simulink model "roachf_1024_bao"  (Simulink 7.5)
settings: Solver=ode45  StartTime=0.0  StopTime=10.0  RelTol=1e-3
undefined symbols (not defined in the file or in its folder): Down, quant, Up
libraries: xbsIndex_r4 x1081, xps_library x49, casper_library_misc x17, casper_library_delays x9, casper_library_sources x4, xbsReplacements_r4 x4, xrbsControl_r4 x1
(part 1 of 11)
settings Model: Creator=zaki  LastModifiedBy=zaki
settings DebuggingCC: StrictBusMsg=Warning

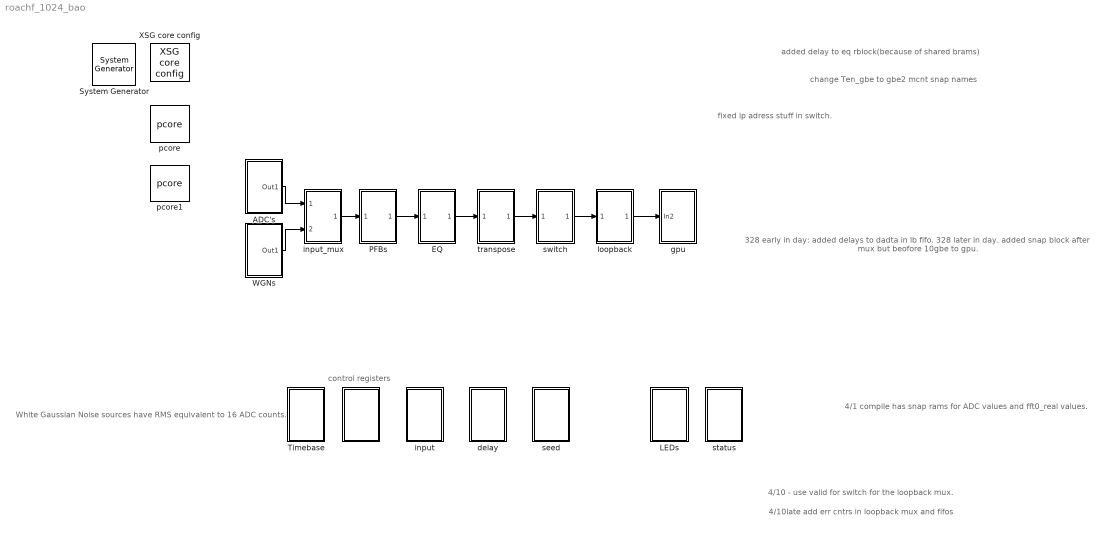
== system roachf_1024_bao ==
  note: White Gaussian Noise
      | sources have RMS
      | equivalent to 16 ADC
      | counts.
  note: fixed ip adress stuff in switch.
  note: 328 early in day: added delays to dadta in lb fifo.
      | 328 later in day. added snap block after mux but beofore
      | 10gbe to gpu.
  note: 4/1 compile has snap rams for ADC values
      | and fft0_real values.
  note: 4/10 - use valid for switch for the loopback mux.
  note: 4/10late add err cntrs in loopback mux and fifos
  note: control registers
  note: added delay to eq rblock(because of shared brams)
  note: change Ten_gbe to gbe2
      | mcnt snap names
  " " : Subsystem
  " System Generator" : xbsIndex_r4/ System Generator  Tag=genX  SystemSampleTime=-1  xilinxfamily=virtex5  part=xc5vsx95t  speed=-1  package=ff1136  synthesis_tool=XST  clock_wrapper=Clock Enables  directory=./roachf_1024_bao/sysgen  proj_type=Project Navigator  Synth_file=XST Defaults  Impl_file=ISE Defaults  testbench=off  simulink_period=1  sysclk_period=6.6667  dcm_input_clock_period=100  incr_netlist=off  trim_vbits=Everywhere in SubSystem  dbl_ovrd=According to Block Masks  core_generation=According to Block Masks  run_coregen=off  deprecated_control=off  eval_field=0  block_type=sysgen
      settings: block_version=10.1.3
  ADC's : Subsystem
  EQ : Subsystem
  LEDs : Subsystem
  PFBs : Subsystem
  Timebase : Subsystem
  WGNs : Subsystem
  XSG core config : xps_library/XSG core config  Tag=xps:xsg  SystemSampleTime=-1  hw_sys=ROACH:sx95t  ibob_linux=off  clk_src=adc0_clk  iBOB_clk_src=adc0_clk  BEE2_ctrl_clk_src=sys_clk  BEE2_usr_clk_src=sys_clk  ROACH_clk_src=adc0_clk  ROACH2_clk_src=adc0_clk  CORR_clk_src=sys_clk  gpio_clk_io_group=iBOB:sma  gpio_clk_bit_index=0  clk_rate=150  sample_period=1  synthesis_tool=XST  mpc_type=powerpc440_ext
  delay : Subsystem
      settings: AttributesFormatString=|
      | Addr 8195
      | 0x2003
  gpu : Subsystem
  input : Subsystem
      settings: AttributesFormatString=|
      | Addr 8194
      | 0x2002
  input_mux : Subsystem
  loopback : Subsystem
  pcore : xps_library/pcore  Tag=xps:pcore  SystemSampleTime=-1  pcore_path=./fft_wideband_real_core2/fft_wideband_real_core2.ngc
  pcore1 : xps_library/pcore  Tag=xps:pcore  SystemSampleTime=-1  pcore_path=./fir_core/fir_core.ngc
  seed : Subsystem
      settings: AttributesFormatString=|
      | Addr 8196
      | 0x2004
  status : Subsystem
  switch : Subsystem
  transpose : Subsystem
  wires:
  PFBs/1(Out1) -> EQ/1(In1)
  EQ/1(Out1) -> transpose/1(In1)
  transpose/1(Out1) -> switch/1(In2)
  switch/1(Out1) -> loopback/1(In1)
  loopback/1(Out1) -> gpu/1(In2)
  WGNs/1(Out1) -> input_mux/2(In2)
  ADC's/1(Out1) -> input_mux/1(In1)
  input_mux/1(Out1) -> PFBs/1(In1)

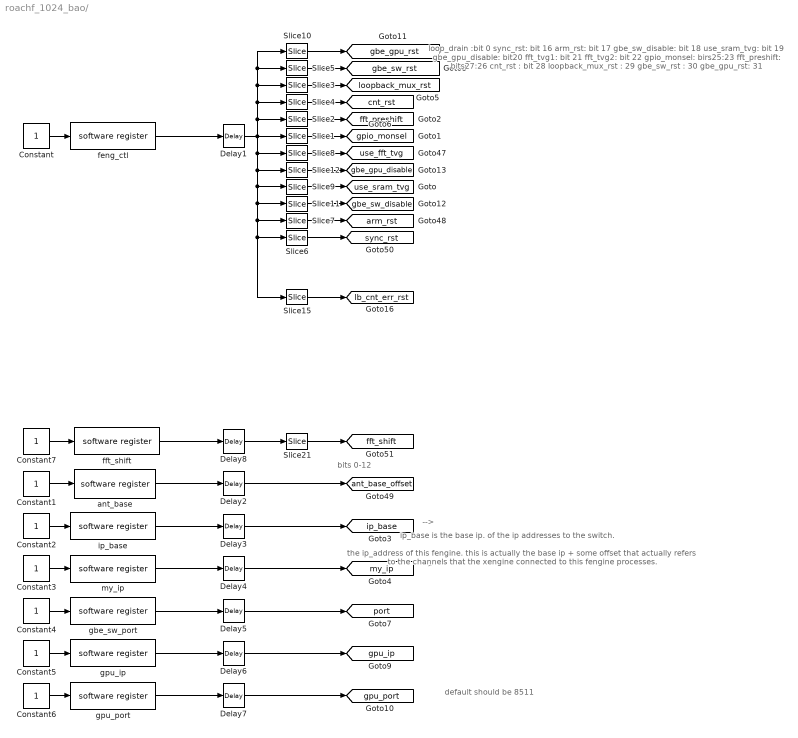
== system roachf_1024_bao/  ==
  note: bits 0-12
  note: default should be 8511
  note: -->
  note: -->
  note: the ip_address of this fengine.
      | this is actually the base ip + some offset
      | that actually refers to the channels that
      | the xengine connected to this fengine
      | processes.
  note: ip_base is the base ip. of
      | the ip addresses to the switch.
  note: loop_drain :bit 0
      |
      | sync_rst: bit 16
      | arm_rst: bit 17
      | gbe_sw_disable: bit 18
      | use_sram_tvg: bit 19
      | gbe_gpu_disable: bit20
      | fft_tvg1: bit 21
      | fft_tvg2: bit 22
      | gpio_monsel: birs25:23
      | fft_preshift: bits27:26
      | cnt_rst : bit 28
      | loopback_mux_rst : 29
      | gbe_sw_rst : 30
      | gbe_gpu_rst: 31
  Constant{,1..7} (8 alike) : Constant
  Delay{1..8} (8 alike) : xbsIndex_r4/Delay  rst=off  infoeditControl=Selection of Reset will increase slice count due to use of real FFs and instead of SRLs  en=off  latency=1  dbl_ovrd=off  reg_retiming=on  block_type=delay
      settings: xl_area=[0, 0, 0, 0, 0, 0, 0]
  Slice1 : xbsIndex_r4/Slice  nbits=3  boolean_output=off  mode=Lower Bit Location + Width  bit1=0  base1=MSB of Input  bit0=23  base0=LSB of Input  dbl_ovrd=off  block_type=slice
      settings: infoedit="Extracts a given range of bits from each input sample and presents it at the output.  The output type is ordinarily unsigned with binary point at zero, but can be Boolean when the slice is one bit wide.<P><P>Hardware notes: In hardware this block costs nothing."  block_version=10.1.3
  Slice10 : xbsIndex_r4/Slice  nbits=16  boolean_output=on  mode=Lower Bit Location + Width  bit1=0  base1=MSB of Input  bit0=31  base0=LSB of Input  dbl_ovrd=off  block_type=slice
      settings: block_version=10.1.3
  Slice11 : xbsIndex_r4/Slice  nbits=1  boolean_output=on  mode=Lower Bit Location + Width  bit1=0  base1=MSB of Input  bit0=18  base0=LSB of Input  dbl_ovrd=off  block_type=slice
      settings: block_version=10.1.3
  Slice12 : xbsIndex_r4/Slice  nbits=1  boolean_output=on  mode=Lower Bit Location + Width  bit1=0  base1=MSB of Input  bit0=20  base0=LSB of Input  dbl_ovrd=off  block_type=slice
      settings: block_version=10.1.3
  Slice15 : xbsIndex_r4/Slice  nbits=1  boolean_output=on  mode=Lower Bit Location + Width  bit1=0  base1=MSB of Input  bit0=2  base0=LSB of Input  dbl_ovrd=off  block_type=slice
      settings: block_version=10.1.3
  Slice2 : xbsIndex_r4/Slice  nbits=2  boolean_output=off  mode=Lower Bit Location + Width  bit1=0  base1=MSB of Input  bit0=26  base0=LSB of Input  dbl_ovrd=off  block_type=slice
      settings: infoedit="Extracts a given range of bits from each input sample and presents it at the output.  The output type is ordinarily unsigned with binary point at zero, but can be Boolean when the slice is one bit wide.<P><P>Hardware notes: In hardware this block costs nothing."  block_version=10.1.3
  Slice21 : xbsIndex_r4/Slice  nbits=13  boolean_output=off  mode=Lower Bit Location + Width  bit1=0  base1=MSB of Input  bit0=0  base0=LSB of Input  dbl_ovrd=off  block_type=slice
      settings: block_version=10.1.3
  Slice3 : xbsIndex_r4/Slice  nbits=16  boolean_output=on  mode=Lower Bit Location + Width  bit1=0  base1=MSB of Input  bit0=29  base0=LSB of Input  dbl_ovrd=off  block_type=slice
      settings: block_version=10.1.3
  Slice4 : xbsIndex_r4/Slice  nbits=16  boolean_output=on  mode=Lower Bit Location + Width  bit1=0  base1=MSB of Input  bit0=28  base0=LSB of Input  dbl_ovrd=off  block_type=slice
      settings: block_version=10.1.3
  Slice5 : xbsIndex_r4/Slice  nbits=16  boolean_output=on  mode=Lower Bit Location + Width  bit1=0  base1=MSB of Input  bit0=30  base0=LSB of Input  dbl_ovrd=off  block_type=slice
      settings: block_version=10.1.3
  Slice6 : xbsIndex_r4/Slice  nbits=1  boolean_output=on  mode=Lower Bit Location + Width  bit1=0  base1=MSB of Input  bit0=16  base0=LSB of Input  dbl_ovrd=off  block_type=slice
      settings: infoedit="Extracts a given range of bits from each input sample and presents it at the output.  The output type is ordinarily unsigned with binary point at zero, but can be Boolean when the slice is one bit wide.<P><P>Hardware notes: In hardware this block costs nothing."  block_version=10.1.3
  Slice7 : xbsIndex_r4/Slice  nbits=1  boolean_output=on  mode=Lower Bit Location + Width  bit1=0  base1=MSB of Input  bit0=17  base0=LSB of Input  dbl_ovrd=off  block_type=slice
      settings: infoedit="Extracts a given range of bits from each input sample and presents it at the output.  The output type is ordinarily unsigned with binary point at zero, but can be Boolean when the slice is one bit wide.<P><P>Hardware notes: In hardware this block costs nothing."  block_version=10.1.3
  Slice8 : xbsIndex_r4/Slice  nbits=2  boolean_output=off  mode=Lower Bit Location + Width  bit1=0  base1=MSB of Input  bit0=21  base0=LSB of Input  dbl_ovrd=off  block_type=slice
      settings: infoedit="Extracts a given range of bits from each input sample and presents it at the output.  The output type is ordinarily unsigned with binary point at zero, but can be Boolean when the slice is one bit wide.<P><P>Hardware notes: In hardware this block costs nothing."  block_version=10.1.3
  Slice9 : xbsIndex_r4/Slice  nbits=1  boolean_output=off  mode=Lower Bit Location + Width  bit1=0  base1=MSB of Input  bit0=19  base0=LSB of Input  dbl_ovrd=off  block_type=slice
      settings: infoedit="Extracts a given range of bits from each input sample and presents it at the output.  The output type is ordinarily unsigned with binary point at zero, but can be Boolean when the slice is one bit wide.<P><P>Hardware notes: In hardware this block costs nothing."  block_version=10.1.3
  ant_base : xps_library/software register  Tag=xps:sw_reg  SystemSampleTime=-1  io_dir=From Processor  arith_type=Unsigned  bitwidth=32  bin_pt=0  sample_period=1  gw_name=roachf_1024_bao_ant_base_user_data_out
  feng_ctl : xps_library/software register  Tag=xps:sw_reg  SystemSampleTime=-1  io_dir=From Processor  arith_type=Unsigned  bitwidth=32  bin_pt=0  sample_period=1  gw_name=roachf_1024_bao_feng_ctl_user_data_out
  fft_shift : xps_library/software register  Tag=xps:sw_reg  SystemSampleTime=-1  io_dir=From Processor  arith_type=Unsigned  bitwidth=32  bin_pt=0  sample_period=1  gw_name=roachf_1024_bao_fft_shift_user_data_out
  gbe_sw_port : xps_library/software register  Tag=xps:sw_reg  SystemSampleTime=-1  io_dir=From Processor  arith_type=Unsigned  bitwidth=32  bin_pt=0  sample_period=1  gw_name=roachf_1024_bao_gbe_sw_port_user_data_out
  gpu_ip : xps_library/software register  Tag=xps:sw_reg  SystemSampleTime=-1  io_dir=From Processor  arith_type=Unsigned  bitwidth=32  bin_pt=0  sample_period=1  gw_name=roachf_1024_bao_gpu_ip_user_data_out
  gpu_port : xps_library/software register  Tag=xps:sw_reg  SystemSampleTime=-1  io_dir=From Processor  arith_type=Unsigned  bitwidth=32  bin_pt=0  sample_period=1  gw_name=roachf_1024_bao_gpu_port_user_data_out
  ip_base : xps_library/software register  Tag=xps:sw_reg  SystemSampleTime=-1  io_dir=From Processor  arith_type=Unsigned  bitwidth=32  bin_pt=0  sample_period=1  gw_name=roachf_1024_bao_ip_base_user_data_out
  my_ip : xps_library/software register  Tag=xps:sw_reg  SystemSampleTime=-1  io_dir=From Processor  arith_type=Unsigned  bitwidth=32  bin_pt=0  sample_period=1  gw_name=roachf_1024_bao_my_ip_user_data_out
  tag scope: ant_base_offset=global, arm_rst=global, cnt_rst=global, fft_preshift=global, fft_shift=global, gbe_gpu_disable=global, gbe_gpu_rst=global, gbe_sw_disable=global, gbe_sw_rst=global, gpio_monsel=global, gpu_ip=global, gpu_port=global, ip_base=global, lb_cnt_err_rst=global, loopback_mux_rst=global, my_ip=global, port=global, sync_rst=global, use_fft_tvg=global, use_sram_tvg=global
  wires:
  Slice15/1 -> [lb_cnt_err_rst]
  Delay8/1 -> Slice21/1
  Constant7/1 -> fft_shift/1
  fft_shift/1 -> Delay8/1
  Slice12/1 -> [gbe_gpu_disable]
  Slice11/1 -> [gbe_sw_disable]
  Slice10/1 -> [gbe_gpu_rst]
  gpu_port/1 -> Delay7/1
  Delay7/1 -> [gpu_port]
  Constant6/1 -> gpu_port/1
  gpu_ip/1 -> Delay6/1
  Delay6/1 -> [gpu_ip]
  Constant5/1 -> gpu_ip/1
  Slice5/1 -> [gbe_sw_rst]
  gbe_sw_port/1 -> Delay5/1
  Delay5/1 -> [port]
  Constant4/1 -> gbe_sw_port/1
  Slice3/1 -> [loopback_mux_rst]
  Slice4/1 -> [cnt_rst]
  my_ip/1 -> Delay4/1
  Delay4/1 -> [my_ip]
  Constant3/1 -> my_ip/1
  ip_base/1 -> Delay3/1
  Delay3/1 -> [ip_base]
  Constant2/1 -> ip_base/1
  Constant1/1 -> ant_base/1
  Constant/1 -> feng_ctl/1
  feng_ctl/1 -> Delay1/1
  Slice2/1 -> [fft_preshift]
  Slice1/1 -> [gpio_monsel]
  Slice9/1 -> [use_sram_tvg]
  Slice7/1 -> [arm_rst]
  Slice6/1 -> [sync_rst]
  Slice21/1 -> [fft_shift]
  Delay1/1 -> Slice10/1, Slice5/1, Slice3/1, Slice4/1, Slice2/1, Slice1/1, Slice12/1, Slice9/1, Slice11/1, Slice15/1, Slice6/1, Slice7/1, Slice8/1
  Slice8/1 -> [use_fft_tvg]
  ant_base/1 -> Delay2/1
  Delay2/1 -> [ant_base_offset]

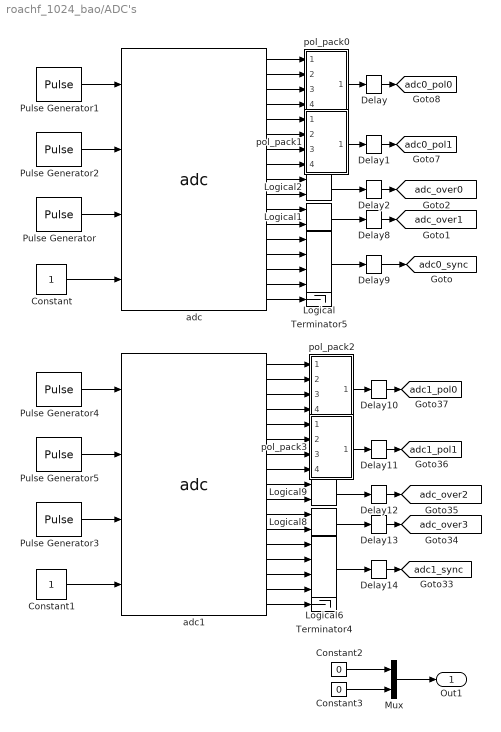
== system roachf_1024_bao/ADC's ==
  Constant : Constant  OutDataType=sfix(16)  OutScaling=2^0  SampleTime=1/4
  Constant1 : Constant  OutDataType=sfix(16)  OutScaling=2^0  SampleTime=1/4
  Constant2 : Constant  Value=0
  Constant3 : Constant  Value=0
  Delay{,1..2,8..14} (10 alike) : xbsIndex_r4/Delay  rst=off  infoeditControl=Selection of Reset will increase slice count due to use of real FFs and instead of SRLs  en=off  latency=1  dbl_ovrd=off  reg_retiming=on  block_type=delay
  Logical : xbsIndex_r4/Logical  logical_function=OR  inputs=4  en=off  latency=0  precision=Full  arith_type=Unsigned  n_bits=16  bin_pt=0  align_bp=on  dbl_ovrd=off  block_type=logical
  Logical{1..2,8..9} (4 alike) : xbsIndex_r4/Logical  logical_function=OR  inputs=2  en=off  latency=0  precision=Full  arith_type=Unsigned  n_bits=16  bin_pt=0  align_bp=on  dbl_ovrd=off  block_type=logical
  Logical6 : xbsIndex_r4/Logical  logical_function=OR  inputs=4  en=off  latency=0  precision=Full  arith_type=Unsigned  n_bits=16  bin_pt=0  align_bp=on  dbl_ovrd=off  block_type=logical
  Mux : Mux  Inputs=2
  Pulse Generator : DiscretePulseGenerator  Amplitude=1  Period=2^8  PulseWidth=1  PhaseDelay=11  SampleTime=1/4
  Pulse Generator1 : DiscretePulseGenerator  Amplitude=0.75  Period=2^10  PulseWidth=1  PhaseDelay=9+13+2^8  SampleTime=1/4
  Pulse Generator2 : DiscretePulseGenerator  Amplitude=0.5  Period=2^10  PulseWidth=1  PhaseDelay=9+14+2^8  SampleTime=1/4
  Pulse Generator3 : DiscretePulseGenerator  Amplitude=1  Period=2^8  PulseWidth=1  PhaseDelay=11  SampleTime=1/4
  Pulse Generator4 : DiscretePulseGenerator  Amplitude=0.75  Period=2^10  PulseWidth=1  PhaseDelay=9+13+2^8  SampleTime=1/4
  Pulse Generator5 : DiscretePulseGenerator  Amplitude=0.5  Period=2^10  PulseWidth=1  PhaseDelay=9+14+2^8  SampleTime=1/4
  Terminator4 : Terminator
  Terminator5 : Terminator
  adc : xps_library/adc  Tag=xps:adc  SystemSampleTime=-1  adc_brd=adc0  adc_clk_rate=600  adc_interleave=off  sample_period=1
  adc1 : xps_library/adc  Tag=xps:adc  SystemSampleTime=-1  adc_brd=adc1  adc_clk_rate=600  adc_interleave=off  sample_period=1
  pol_pack0 : Subsystem
  pol_pack1 : Subsystem
  pol_pack2 : Subsystem
  pol_pack3 : Subsystem
  Out1 : Outport  OutDataType=sfix(16)  OutScaling=2^0
  tag scope: adc0_pol0=global, adc0_pol1=global, adc0_sync=global, adc1_pol0=global, adc1_pol1=global, adc1_sync=global, adc_over0=global, adc_over1=global, adc_over2=global, adc_over3=global
  wires:
  Delay/1 -> [adc0_pol0]
  Delay1/1 -> [adc0_pol1]
  Delay2/1 -> [adc_over0]
  Delay8/1 -> [adc_over1]
  Delay9/1 -> [adc0_sync]
  Delay10/1 -> [adc1_pol0]
  Delay11/1 -> [adc1_pol1]
  Delay12/1 -> [adc_over2]
  Delay13/1 -> [adc_over3]
  Delay14/1 -> [adc1_sync]
  pol_pack2/1(Out1) -> Delay10/1
  adc1/4 -> pol_pack2/4(In4)
  adc1/3 -> pol_pack2/3(In3)
  adc1/2 -> pol_pack2/2(In2)
  adc1/1 -> pol_pack2/1(In1)
  pol_pack3/1(Out1) -> Delay11/1
  adc1/8 -> pol_pack3/4(In4)
  adc1/7 -> pol_pack3/3(In3)
  adc1/6 -> pol_pack3/2(In2)
  adc1/5 -> pol_pack3/1(In1)
  Logical8/1 -> Delay13/1
  Logical9/1 -> Delay12/1
  adc1/12 -> Logical8/2
  adc1/11 -> Logical8/1
  adc1/10 -> Logical9/2
  adc1/9 -> Logical9/1
  adc1/17 -> Terminator4/1
  Logical6/1 -> Delay14/1
  adc1/13 -> Logical6/1
  adc1/14 -> Logical6/2
  adc1/15 -> Logical6/3
  adc1/16 -> Logical6/4
  adc/17 -> Terminator5/1
  adc/16 -> Logical/4
  adc/15 -> Logical/3
  adc/14 -> Logical/2
  adc/13 -> Logical/1
  adc/12 -> Logical1/2
  adc/11 -> Logical1/1
  adc/10 -> Logical2/2
  adc/9 -> Logical2/1
  adc/8 -> pol_pack1/4(In4)
  adc/7 -> pol_pack1/3(In3)
  adc/6 -> pol_pack1/2(In2)
  adc/5 -> pol_pack1/1(In1)
  adc/4 -> pol_pack0/4(In4)
  adc/3 -> pol_pack0/3(In3)
  adc/2 -> pol_pack0/2(In2)
  adc/1 -> pol_pack0/1(In1)
  Logical1/1 -> Delay8/1
  pol_pack0/1(Out1) -> Delay/1
  pol_pack1/1(Out1) -> Delay1/1
  Logical2/1 -> Delay2/1
  Logical/1 -> Delay9/1
  Constant1/1 -> adc1/4
  Pulse Generator5/1 -> adc1/2
  Pulse Generator4/1 -> adc1/1
  Pulse Generator3/1 -> adc1/3
  Constant/1 -> adc/4
  Pulse Generator2/1 -> adc/2
  Pulse Generator1/1 -> adc/1
  Pulse Generator/1 -> adc/3
  Constant3/1 -> Mux/2
  Constant2/1 -> Mux/1
  Mux/1 -> Out1/1

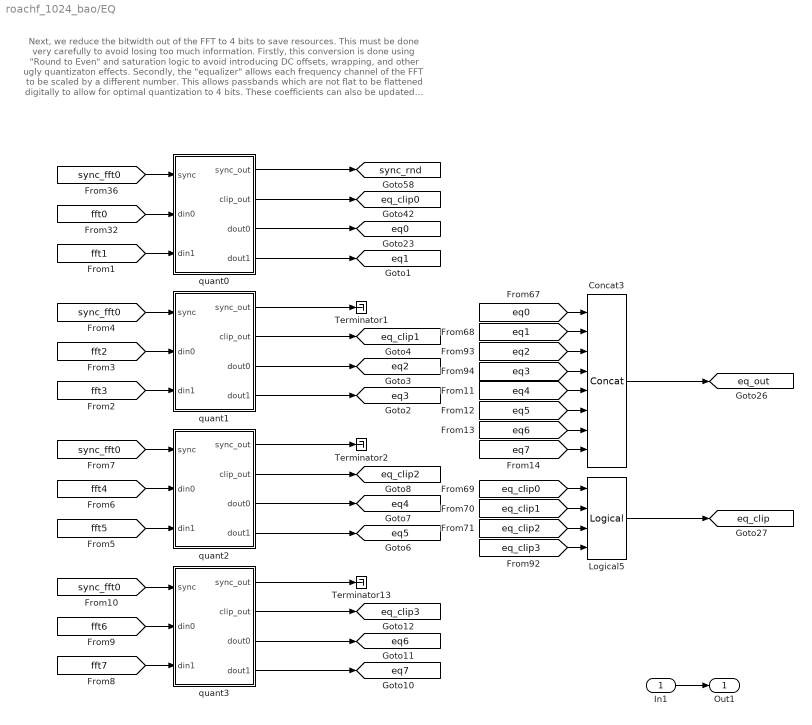
== system roachf_1024_bao/EQ ==
  note: Next, we reduce the bitwidth out of the FFT to 4 bits to save resources.
      | This must be done very carefully to avoid losing too much information.
      | Firstly, this conversion is done using "Round to Even" and saturation
      | logic to avoid introducing DC offsets, wrapping, and other ugly quantizaton
      | effects.  Secondly, the "equalizer" allows each frequency channel of the
      | FFT to be scaled by a different number.  This allows passbands which are
      | not flat to be flattened digitally to allow for optimal quantization to 4 bits.
      | These coefficients can also be updated dynamically for gain control.
      | Coefficients can be dynamically written into the "equalizer" by
      | specifying the channel ("coeff_addr") and the value of the
      | coefficient ("coeff"), and then using "coeff_en" to write the
      | new coefficient into the equalization table.
  In1 : Inport
  Concat3 : xbsIndex_r4/Concat  num_inputs=8  dbl_ovrd=off  block_type=concat
      settings: block_version=10.1.3
  Logical5 : xbsIndex_r4/Logical  logical_function=OR  inputs=4  en=off  latency=0  precision=Full  arith_type=Unsigned  n_bits=8  bin_pt=2  align_bp=on  dbl_ovrd=off  block_type=logical
      settings: xl_area=[0, 0, 0, 0, 0, 0, 0]
  Terminator1 : Terminator
  Terminator13 : Terminator
  Terminator2 : Terminator
  quant0 : Subsystem
  quant1 : Subsystem
  quant2 : Subsystem
  quant3 : Subsystem
  Out1 : Outport
  tag scope: eq0=global, eq1=global, eq2=global, eq3=global, eq4=global, eq5=global, eq6=global, eq7=global, eq_clip0=global, eq_clip1=global, eq_clip2=global, eq_clip3=global, eq_clip=global, eq_out=global, sync_rnd=global
  wires:
  Logical5/1 -> [eq_clip]
  Concat3/1 -> [eq_out]
  [eq_clip0] -> Logical5/1
  [eq_clip1] -> Logical5/2
  [eq_clip2] -> Logical5/3
  [eq_clip3] -> Logical5/4
  [eq0] -> Concat3/1
  [eq1] -> Concat3/2
  [eq2] -> Concat3/3
  [eq3] -> Concat3/4
  In1/1 -> Out1/1
  [sync_fft0] -> quant0/1(sync)
  [fft0] -> quant0/2(din0)
  [fft1] -> quant0/3(din1)
  quant0/1(sync_out) -> [sync_rnd]
  quant0/2(clip_out) -> [eq_clip0]
  quant0/3(dout0) -> [eq0]
  quant0/4(dout1) -> [eq1]
  [sync_fft0] -> quant1/1(sync)
  [fft2] -> quant1/2(din0)
  [fft3] -> quant1/3(din1)
  [sync_fft0] -> quant2/1(sync)
  [fft4] -> quant2/2(din0)
  [fft5] -> quant2/3(din1)
  [sync_fft0] -> quant3/1(sync)
  [fft6] -> quant3/2(din0)
  [fft7] -> quant3/3(din1)
  quant1/1(sync_out) -> Terminator1/1
  quant1/2(clip_out) -> [eq_clip1]
  quant1/3(dout0) -> [eq2]
  quant1/4(dout1) -> [eq3]
  quant2/1(sync_out) -> Terminator2/1
  quant2/2(clip_out) -> [eq_clip2]
  quant2/3(dout0) -> [eq4]
  quant2/4(dout1) -> [eq5]
  quant3/1(sync_out) -> Terminator13/1
  quant3/2(clip_out) -> [eq_clip3]
  quant3/3(dout0) -> [eq6]
  quant3/4(dout1) -> [eq7]
  [eq4] -> Concat3/5
  [eq5] -> Concat3/6
  [eq6] -> Concat3/7
  [eq7] -> Concat3/8

== system roachf_1024_bao/LEDs ==
  Delay{,1..2,4..6} (6 alike) : xbsIndex_r4/Delay  rst=off  infoeditControl=Selection of Reset will increase slice count due to use of real FFs and instead of SRLs  en=off  latency=1  dbl_ovrd=off  reg_retiming=off  block_type=delay
  Terminator2 : Terminator
  Terminator27 : Terminator
  Terminator3 : Terminator
  led1_arm : xps_library/gpio  Tag=xps:gpio  SystemSampleTime=-1  io_group=ROACH:led  io_dir=out  arith_type=Boolean  bitwidth=1  bin_pt=0  bit_index=0  sample_period=1  use_single_ended=off  use_ddr=off  reg_iob=on  reg_clk_phase=0  termination=None
      link override convert: arith_type=Boolean  n_bits=1  bin_pt=0
  led2_sync : xps_library/gpio  Tag=xps:gpio  SystemSampleTime=-1  io_group=ROACH:led  io_dir=out  arith_type=Boolean  bitwidth=1  bin_pt=0  bit_index=1  sample_period=1  use_single_ended=off  use_ddr=off  reg_iob=on  reg_clk_phase=0  termination=None
      link override convert: arith_type=Boolean  n_bits=1  bin_pt=0
  led4_eq_clip : xps_library/gpio  Tag=xps:gpio  SystemSampleTime=-1  io_group=ROACH:led  io_dir=out  arith_type=Boolean  bitwidth=1  bin_pt=0  bit_index=2  sample_period=1  use_single_ended=off  use_ddr=off  reg_iob=on  reg_clk_phase=0  termination=None
      link override convert: arith_type=Boolean  n_bits=1  bin_pt=0
  pulse_ext2 : Subsystem  mask{pulse_len=2^23}
      mask prompts: pulse_len "Length of Pulse"
      mask init:
      | bits = ceil(log2(pulse_len+1));
  pulse_ext4 : Subsystem  mask{pulse_len=2^18}
      mask prompts: pulse_len "Length of Pulse"
      mask init:
      | bits = ceil(log2(pulse_len+1));
  wires:
  pulse_ext2/1(out) -> Delay5/1
  [sync_gen] -> Delay1/1
  [armed] -> Delay/1
  pulse_ext4/1(out) -> Delay6/1
  [eq_clip] -> Delay2/1
  led1_arm/1 -> Terminator27/1
  led4_eq_clip/1 -> Terminator2/1
  led2_sync/1 -> Terminator3/1
  Delay/1 -> Delay4/1
  Delay2/1 -> pulse_ext4/1(in)
  Delay1/1 -> pulse_ext2/1(in)
  Delay6/1 -> led4_eq_clip/1
  Delay5/1 -> led2_sync/1
  Delay4/1 -> led1_arm/1

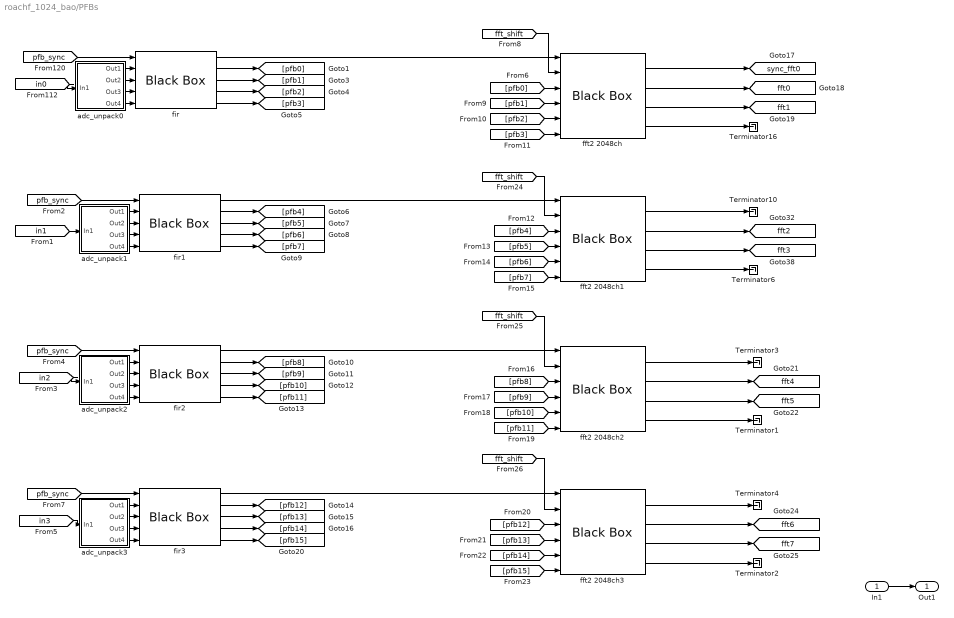
== system roachf_1024_bao/PFBs ==
  In1 : Inport
  Terminator{1..4,6,10,16} (7 alike) : Terminator
  adc_unpack0 : Subsystem
  adc_unpack1 : Subsystem
  adc_unpack2 : Subsystem
  adc_unpack3 : Subsystem
  fft2 2048ch{,1..3} (4 alike) : xbsIndex_r4/Black Box  init_code=fft_wideband_real_core2_config  sim_method=Inactive  verbose=off  block_type=blackbox2
  fir{,1..3} (4 alike) : xbsIndex_r4/Black Box  init_code=fir_core_config  sim_method=Inactive  verbose=off  block_type=blackbox2
  Out1 : Outport
  tag scope: fft0=global, fft1=global, fft2=global, fft3=global, fft4=global, fft5=global, fft6=global, fft7=global, sync_fft0=global
  wires:
  [pfb_sync] -> fir/1
  In1/1 -> Out1/1
  fir/1 -> fft2 2048ch/1
  [in0] -> adc_unpack0/1(In1)
  adc_unpack0/1(Out1) -> fir/2
  adc_unpack0/2(Out2) -> fir/3
  adc_unpack0/3(Out3) -> fir/4
  adc_unpack0/4(Out4) -> fir/5
  [pfb_sync] -> fir1/1
  [in1] -> adc_unpack1/1(In1)
  adc_unpack1/1(Out1) -> fir1/2
  adc_unpack1/2(Out2) -> fir1/3
  adc_unpack1/3(Out3) -> fir1/4
  adc_unpack1/4(Out4) -> fir1/5
  [pfb_sync] -> fir2/1
  [in2] -> adc_unpack2/1(In1)
  adc_unpack2/1(Out1) -> fir2/2
  adc_unpack2/2(Out2) -> fir2/3
  adc_unpack2/3(Out3) -> fir2/4
  adc_unpack2/4(Out4) -> fir2/5
  [pfb_sync] -> fir3/1
  [in3] -> adc_unpack3/1(In1)
  adc_unpack3/1(Out1) -> fir3/2
  adc_unpack3/2(Out2) -> fir3/3
  adc_unpack3/3(Out3) -> fir3/4
  adc_unpack3/4(Out4) -> fir3/5
  [fft_shift] -> fft2 2048ch/2
  fir/2 -> [pfb0]
  fir/3 -> [pfb1]
  fir/4 -> [pfb2]
  fir/5 -> [pfb3]
  fir1/2 -> [pfb4]
  fir1/3 -> [pfb5]
  fir1/4 -> [pfb6]
  fir1/5 -> [pfb7]
  fir2/2 -> [pfb8]
  fir2/3 -> [pfb9]
  fir2/4 -> [pfb10]
  fir2/5 -> [pfb11]
  fir1/1 -> fft2 2048ch1/1
  fir3/2 -> [pfb12]
  fir3/3 -> [pfb13]
  fir3/4 -> [pfb14]
  fir3/5 -> [pfb15]
  [pfb0] -> fft2 2048ch/3
  fir3/1 -> fft2 2048ch3/1
  fir2/1 -> fft2 2048ch2/1
  [pfb3] -> fft2 2048ch/6
  [pfb2] -> fft2 2048ch/5
  [pfb1] -> fft2 2048ch/4
  [pfb7] -> fft2 2048ch1/6
  [pfb6] -> fft2 2048ch1/5
  [pfb5] -> fft2 2048ch1/4
  [pfb4] -> fft2 2048ch1/3
  [pfb8] -> fft2 2048ch2/3
  [pfb9] -> fft2 2048ch2/4
  [pfb10] -> fft2 2048ch2/5
  [pfb11] -> fft2 2048ch2/6
  [pfb12] -> fft2 2048ch3/3
  [pfb14] -> fft2 2048ch3/5
  [pfb13] -> fft2 2048ch3/4
  [pfb15] -> fft2 2048ch3/6
  [fft_shift] -> fft2 2048ch1/2
  [fft_shift] -> fft2 2048ch2/2
  [fft_shift] -> fft2 2048ch3/2
  fft2 2048ch/1 -> [sync_fft0]
  fft2 2048ch/2 -> [fft0]
  fft2 2048ch/3 -> [fft1]
  fft2 2048ch/4 -> Terminator16/1
  fft2 2048ch2/2 -> [fft4]
  fft2 2048ch2/3 -> [fft5]
  fft2 2048ch2/4 -> Terminator1/1
  fft2 2048ch3/2 -> [fft6]
  fft2 2048ch3/3 -> [fft7]
  fft2 2048ch3/4 -> Terminator2/1
  fft2 2048ch1/1 -> Terminator10/1
  fft2 2048ch1/2 -> [fft2]
  fft2 2048ch1/3 -> [fft3]
  fft2 2048ch1/4 -> Terminator6/1
  fft2 2048ch2/1 -> Terminator3/1
  fft2 2048ch3/1 -> Terminator4/1

== system roachf_1024_bao/Timebase ==
  note: This circuit implements a schem for synchronizing multiple roachs
      | to a 150MHz clock. A 1PPS is supplied to the sync input for the
      | iADCs. An arm signal is transmitted to the ROACHS which gets
      | released at the next sync pulse.  Note that the sync pulse
      | generator needs to be a multiple of the base sync pulse.
      | fftchannels/simultaneous inputs *  lcm(order of reorders) * pfb taps.
      |
      | base syncpulse = lcm(2,2,2,3,9)*512*4 = 36864.
      | This sync pulse generates a pulse every 9*2^24 clocs.
      | which at 150MHz is roughly 1 second.
  Logical7 : xbsIndex_r4/Logical  logical_function=OR  inputs=3  en=off  latency=1  precision=Full  arith_type=Unsigned  n_bits=8  bin_pt=2  align_bp=on  dbl_ovrd=off  block_type=logical
      settings: xl_area=[0, 0, 0, 0, 0, 0, 0]
  sync_gen : Subsystem
  tag scope: armed=global, mrst=global, sync_gen=global
  wires:
  sync_gen/1(sync) -> [sync_gen]
  sync_gen/2(mrst) -> [mrst]
  [arm_rst] -> sync_gen/2(arm)
  [sync_rst] -> Logical7/2
  sync_gen/3(armed) -> [armed]
  Logical7/1 -> sync_gen/1(rst)
  [adc0_sync] -> Logical7/1
  [adc1_sync] -> Logical7/3

== system roachf_1024_bao/WGNs ==
  Constant : Constant  Value=0
  Constant2 : Constant  Value=0
  Delay1 : xbsIndex_r4/Delay  rst=off  infoeditControl=Selection of Reset will increase slice count due to use of real FFs and instead of SRLs  en=off  latency=3  dbl_ovrd=off  reg_retiming=on  block_type=delay
  Delay2 : xbsIndex_r4/Delay  rst=off  infoeditControl=Selection of Reset will increase slice count due to use of real FFs and instead of SRLs  en=off  latency=3  dbl_ovrd=off  reg_retiming=on  block_type=delay
  Mux : Mux  Inputs=2
  noise0 : Subsystem
  noise1 : Subsystem
  noise3 : Subsystem
  noise4 : Subsystem
  pol_pack0 : Subsystem
  pol_pack1 : Subsystem
  Out1 : Outport  OutDataType=sfix(16)  OutScaling=2^0
  tag scope: n0=global, n1=global
  wires:
  [seed_ld] -> noise1/2(ld)
  [seed_ld] -> noise3/2(ld)
  [seed_ld] -> noise4/2(ld)
  [seed_ld] -> noise0/2(ld)
  [seed1] -> noise1/1(seed)
  [seed2] -> noise3/1(seed)
  [seed3] -> noise4/1(seed)
  [seed0] -> noise0/1(seed)
  Constant2/1 -> Mux/2
  Constant/1 -> Mux/1
  Mux/1 -> Out1/1
  noise0/1(n1) -> pol_pack0/1(In1)
  noise0/2(n2) -> pol_pack0/2(In2)
  noise1/1(n1) -> pol_pack0/3(In3)
  noise1/2(n2) -> pol_pack0/4(In4)
  pol_pack0/1(Out1) -> Delay2/1
  noise3/1(n1) -> pol_pack1/1(In1)
  noise3/2(n2) -> pol_pack1/2(In2)
  noise4/1(n1) -> pol_pack1/3(In3)
  noise4/2(n2) -> pol_pack1/4(In4)
  pol_pack1/1(Out1) -> Delay1/1
  Delay1/1 -> [n1]
  Delay2/1 -> [n0]

== system roachf_1024_bao/delay ==
  BitBasher : xbsIndex_r4/BitBasher  bitexpr=|  display_expr=off  sr_1=1  arith_type1=Unsigned  bin_pt1=0  sr_2=2  arith_type2=Unsigned  bin_pt2=0  sr_3=3  arith_type3=Unsigned  bin_pt3=0  sr_4=4  arith_type4=Unsigned  bin_pt4=0  dbl_ovrd=off  block_type=bitbasher
      | <html><head><meta name="qrichtext" content="1" /><style type="text/css">
      | p, li { white-space: pre-wrap; }
      | </style></head><body style=" font-family:'MS Shell Dlg 2'; font-size:8.25pt; font-weight:400; font-style:normal;">
      | <p style=" margin-top:12px; margin-bottom:12px; margin-left:0px; margin-right:0px; -qt-block-indent:0; text-indent:0px; font-family:'MS Shell Dlg'; font-size:8pt;">delay0={delay[3:0]}<br />delay1={delay[7:4]}<br />delay2={delay[11:8]}<br />delay3={delay[15:12]}</p></body></html>
      settings: block_version=10.1.3
  BitBasher1 : xbsIndex_r4/BitBasher  bitexpr=|  display_expr=off  sr_1=1  arith_type1=Unsigned  bin_pt1=0  sr_2=2  arith_type2=Unsigned  bin_pt2=0  sr_3=3  arith_type3=Unsigned  bin_pt3=0  sr_4=4  arith_type4=Unsigned  bin_pt4=0  dbl_ovrd=off  block_type=bitbasher
      | <html><head><meta name="qrichtext" content="1" /><style type="text/css">
      | p, li { white-space: pre-wrap; }
      | </style></head><body style=" font-family:'MS Shell Dlg 2'; font-size:8.25pt; font-weight:400; font-style:normal;">
      | <p style=" margin-top:12px; margin-bottom:12px; margin-left:0px; margin-right:0px; -qt-block-indent:0; text-indent:0px; font-family:'MS Shell Dlg'; font-size:8pt;">delay4={delay[19:16]}<br />delay5={delay[23:20]}<br />delay6={delay[27:24]}<br />delay7={delay[31:28]}</p></body></html>
      settings: block_version=10.1.3
  values : xps_library/software register  Tag=xps:sw_reg  SystemSampleTime=-1  io_dir=From Processor  arith_type=Unsigned  bitwidth=32  bin_pt=0  sample_period=1  gw_name=roachf_1024_bao_delay_values_user_data_out
  tag scope: delay0=global, delay1=global, delay2=global, delay3=global, delay4=global, delay5=global, delay6=global, delay7=global
  wires:
  values/1 -> BitBasher1/1, BitBasher/1
  BitBasher1/4 -> [delay7]
  BitBasher1/3 -> [delay6]
  BitBasher1/2 -> [delay5]
  BitBasher1/1 -> [delay4]
  BitBasher/4 -> [delay3]
  BitBasher/3 -> [delay2]
  BitBasher/2 -> [delay1]
  BitBasher/1 -> [delay0]

== system roachf_1024_bao/gpu ==
  note: data comes in directly from the loopback musx into the ten gbe core
  In2 : Inport
  Constant2 : xbsIndex_r4/Constant  const=0  gui_display_data_type=Fixed-point  arith_type=Boolean  n_bits=16  bin_pt=14  preci_type=Single  exp_width=8  frac_width=24  explicit_period=on  period=1  equ=P=C  opselect=C  inp2=PCIN>>17  opr=+  inp1=P  carry=CIN  dbl_ovrd=off  block_type=constant
      settings: block_version=11.4
  Delay1 : xbsIndex_r4/Delay  rst=off  infoeditControl=Selection of Reset will increase slice count due to use of real FFs and instead of SRLs  en=off  latency=2  dbl_ovrd=off  reg_retiming=off  block_type=delay
  Delay2 : xbsIndex_r4/Delay  rst=off  infoeditControl=Selection of Reset will increase slice count due to use of real FFs and instead of SRLs  en=off  latency=2  dbl_ovrd=off  reg_retiming=off  block_type=delay
  Delay3 : xbsIndex_r4/Delay  rst=off  infoeditControl=Selection of Reset will increase slice count due to use of real FFs and instead of SRLs  en=off  latency=2  dbl_ovrd=off  reg_retiming=off  block_type=delay
  Inverter : xbsIndex_r4/Inverter  en=off  latency=0  dbl_ovrd=off  block_type=inv
      settings: block_version=11.4
  Logical : xbsIndex_r4/Logical  logical_function=AND  inputs=2  en=off  latency=0  precision=Full  arith_type=Unsigned  n_bits=16  bin_pt=0  align_bp=on  dbl_ovrd=off  block_type=logical
      settings: block_version=11.4
  Terminator : Terminator
  gbe2 : xps_library/ten_Gbe_v2  Tag=xps:tengbe_v2  SystemSampleTime=-1  port=2  rx_dist_ram=off  large_frames=on  show_param=on  pre_emph=3  swing=800  fab_en=off  fab_mac=hex2dec('123456780000')  fab_ip=192*(2^24) + 168*(2^16) + 5*(2^8) + 20*(2^0)  fab_udp=10000  fab_gate=1  cpu_rx_en=off  cpu_tx_en=on
  tag scope: gbe_gpu_led_rx=global, gbe_gpu_led_tx=global, gbe_gpu_led_up=global, gbe_gpu_rx_data=global, gbe_gpu_rx_eof=global, gbe_gpu_rx_ip=global, gbe_gpu_rx_port=global, gbe_gpu_rx_size=global, gbe_gpu_rx_valid=global, gbe_gpu_tx_ack=global
  wires:
  In2/1 -> Terminator/1
  [lb_mux_valid] -> Delay1/1
  [gbe_gpu_disable] -> Inverter/1
  Inverter/1 -> Logical/1
  Logical/1 -> gbe2/3
  Delay1/1 -> Logical/2
  [gbe_gpu_rst] -> gbe2/1
  [lb_mux_data] -> Delay2/1
  Delay2/1 -> gbe2/2
  [gpu_ip] -> gbe2/4
  Delay3/1 -> gbe2/6
  [gpu_port] -> gbe2/5
  [lb_mux_eof] -> Delay3/1
  Constant2/1 -> gbe2/8, gbe2/7
  gbe2/1 -> [gbe_gpu_led_up]
  gbe2/2 -> [gbe_gpu_led_rx]
  gbe2/3 -> [gbe_gpu_led_tx]
  gbe2/4 -> [gbe_gpu_tx_ack]
  gbe2/6 -> [gbe_gpu_rx_data]
  gbe2/7 -> [gbe_gpu_rx_valid]
  gbe2/8 -> [gbe_gpu_rx_ip]
  gbe2/9 -> [gbe_gpu_rx_port]
  gbe2/10 -> [gbe_gpu_rx_eof]
  gbe2/12 -> [gbe_gpu_rx_size]

== system roachf_1024_bao/input ==
  BitBasher : xbsIndex_r4/BitBasher  bitexpr=|  display_expr=off  sr_1=1  arith_type1=Unsigned  bin_pt1=0  sr_2=2  arith_type2=Unsigned  bin_pt2=0  sr_3=3  arith_type3=Unsigned  bin_pt3=0  sr_4=4  arith_type4=Unsigned  bin_pt4=0  dbl_ovrd=off  block_type=bitbasher
      | <html><head><meta name="qrichtext" content="1" /><style type="text/css">
      | p, li { white-space: pre-wrap; }
      | </style></head><body style=" font-family:'MS Shell Dlg 2'; font-size:8.25pt; font-weight:400; font-style:normal;">
      | <p style=" margin-top:12px; margin-bottom:12px; margin-left:0px; margin-right:0px; -qt-block-indent:0; text-indent:0px; font-family:'MS Shell Dlg'; font-size:8pt;">insel0={insel[1:0]}<br />insel1={insel[5:4]}<br />insel2={insel[9:8]}<br />insel3={insel[13:12]}</p></body></html>
      settings: block_version=10.1.3
  BitBasher1 : xbsIndex_r4/BitBasher  bitexpr=|  display_expr=off  sr_1=1  arith_type1=Unsigned  bin_pt1=0  sr_2=2  arith_type2=Unsigned  bin_pt2=0  sr_3=3  arith_type3=Unsigned  bin_pt3=0  sr_4=4  arith_type4=Unsigned  bin_pt4=0  dbl_ovrd=off  block_type=bitbasher
      | <html><head><meta name="qrichtext" content="1" /><style type="text/css">
      | p, li { white-space: pre-wrap; }
      | </style></head><body style=" font-family:'MS Shell Dlg 2'; font-size:8.25pt; font-weight:400; font-style:normal;">
      | <p style=" margin-top:12px; margin-bottom:12px; margin-left:0px; margin-right:0px; -qt-block-indent:0; text-indent:0px; font-family:'MS Shell Dlg'; font-size:8pt;">insel4={insel[17:16]}<br />insel5={insel[21:20]}<br />insel6={insel[25:24]}<br />insel7={insel[29:28]}</p></body></html>
      settings: block_version=10.1.3
  selector : xps_library/software register  Tag=xps:sw_reg  SystemSampleTime=-1  io_dir=From Processor  arith_type=Unsigned  bitwidth=32  bin_pt=0  sample_period=1  gw_name=roachf_1024_bao_input_selector_user_data_out
  tag scope: insel0=global, insel1=global, insel2=global, insel3=global, insel4=global, insel5=global, insel6=global, insel7=global
  wires:
  selector/1 -> BitBasher1/1, BitBasher/1
  BitBasher1/4 -> [insel7]
  BitBasher1/3 -> [insel6]
  BitBasher1/2 -> [insel5]
  BitBasher1/1 -> [insel4]
  BitBasher/4 -> [insel3]
  BitBasher/3 -> [insel2]
  BitBasher/2 -> [insel1]
  BitBasher/1 -> [insel0]

== system roachf_1024_bao/input_mux ==
  In1 : Inport  OutDataType=sfix(16)  OutScaling=2^0
  In2 : Inport  Port=2  OutDataType=sfix(16)  OutScaling=2^0
  Delay : xbsIndex_r4/Delay  rst=off  infoeditControl=Selection of Reset will increase slice count due to use of real FFs and instead of SRLs  en=off  latency=2  dbl_ovrd=off  reg_retiming=off  block_type=delay
  Delay{1..5} (5 alike) : xbsIndex_r4/Delay  rst=off  infoeditControl=Selection of Reset will increase slice count due to use of real FFs and instead of SRLs  en=off  latency=1  dbl_ovrd=off  reg_retiming=on  block_type=delay
  Terminator : Terminator
  muxin0 : Subsystem
  muxin1 : Subsystem
  muxin2 : Subsystem
  muxin3 : Subsystem
  Out1 : Outport
  tag scope: in0=global, in1=global, in2=global, in3=global, pfb_sync=global
  wires:
  In2/1 -> Terminator/1
  In1/1 -> Out1/1
  Delay/1 -> Delay5/1
  [sync_gen] -> Delay/1
  muxin3/1(out) -> Delay4/1
  muxin2/1(out) -> Delay3/1
  muxin1/1(out) -> Delay2/1
  [delay3] -> muxin3/5(delay)
  [adc1_pol1] -> muxin3/2(adc)
  [insel3] -> muxin3/1(sel)
  [delay2] -> muxin2/5(delay)
  [n1] -> muxin2/4(n1), muxin3/4(n1)
  [n0] -> muxin2/3(n0), muxin3/3(n0)
  [adc1_pol0] -> muxin2/2(adc)
  [insel2] -> muxin2/1(sel)
  [delay1] -> muxin1/5(delay)
  [adc0_pol1] -> muxin1/2(adc)
  [insel1] -> muxin1/1(sel)
  muxin0/1(out) -> Delay1/1
  [delay0] -> muxin0/5(delay)
  [n1] -> muxin1/4(n1), muxin0/4(n1)
  [n0] -> muxin1/3(n0), muxin0/3(n0)
  [adc0_pol0] -> muxin0/2(adc)
  [insel0] -> muxin0/1(sel)
  Delay1/1 -> [in0]
  Delay2/1 -> [in1]
  Delay3/1 -> [in2]
  Delay4/1 -> [in3]
  Delay5/1 -> [pfb_sync]

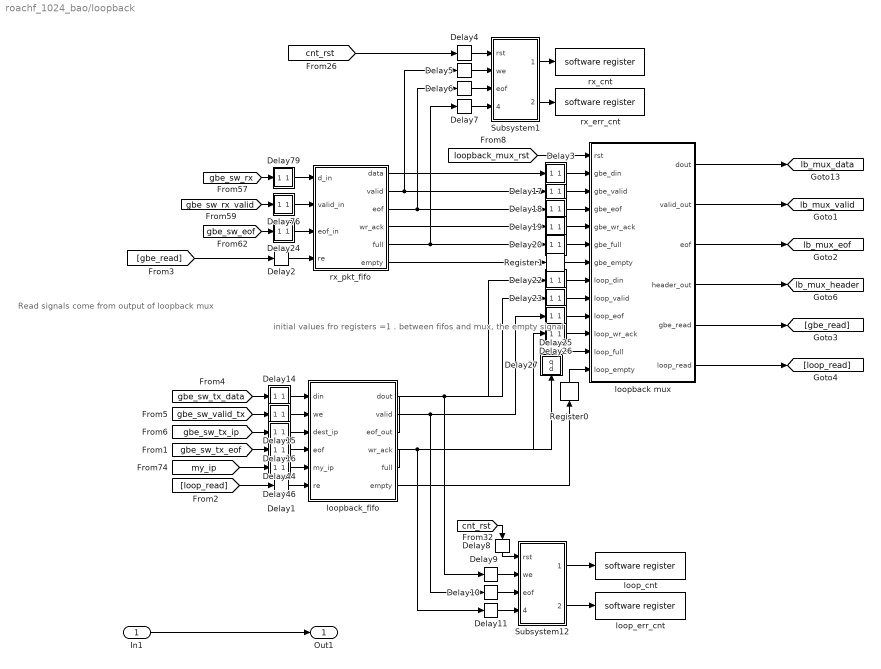
== system roachf_1024_bao/loopback ==
  note: Read signals come from output of
      | loopback mux
  note: initial values fro registers =1 .
      | between fifos and mux, the
      | empty signal
  In1 : Inport
  Delay1 : xbsIndex_r4/Delay  rst=off  infoeditControl=Selection of Reset will increase slice count due to use of real FFs and instead of SRLs  en=off  latency=2  dbl_ovrd=off  reg_retiming=off  block_type=delay
  Delay{4..11} (8 alike) : xbsIndex_r4/Delay  rst=off  infoeditControl=Selection of Reset will increase slice count due to use of real FFs and instead of SRLs  en=off  latency=1  dbl_ovrd=off  reg_retiming=off  block_type=delay
  Delay14 : Subsystem  AncestorBlock=casper_library/Delays/pipeline  mask(pipeline){latency=2}
      mask help:
      | An explicitly laid-out delay line to avoid mapping to SRL16s
      | for use in pipelining to help achieve timing closure.
      mask init:
      | pipeline_init(gcb, 'latency', latency);
      mask Display:
      | port_label('input', 1, 'd');
      | port_label('output', 1, 'q');
      | disp(['Z^-', num2str(latency)]);
  Delay15 : Subsystem  AncestorBlock=casper_library/Delays/pipeline  mask(pipeline){latency=2}
      mask help:
      | An explicitly laid-out delay line to avoid mapping to SRL16s
      | for use in pipelining to help achieve timing closure.
      mask init:
      | pipeline_init(gcb, 'latency', latency);
      mask Display:
      | port_label('input', 1, 'd');
      | port_label('output', 1, 'q');
      | disp(['Z^-', num2str(latency)]);
  Delay16 : Subsystem  AncestorBlock=casper_library/Delays/pipeline  mask(pipeline){latency=2}
      mask help:
      | An explicitly laid-out delay line to avoid mapping to SRL16s
      | for use in pipelining to help achieve timing closure.
      mask init:
      | pipeline_init(gcb, 'latency', latency);
      mask Display:
      | port_label('input', 1, 'd');
      | port_label('output', 1, 'q');
      | disp(['Z^-', num2str(latency)]);
  Delay17 : Subsystem  AncestorBlock=casper_library/Delays/pipeline  mask(pipeline){latency=1}
      mask help:
      | An explicitly laid-out delay line to avoid mapping to SRL16s
      | for use in pipelining to help achieve timing closure.
      mask init:
      | pipeline_init(gcb, 'latency', latency);
      mask Display:
      | port_label('input', 1, 'd');
      | port_label('output', 1, 'q');
      | disp(['Z^-', num2str(latency)]);
  Delay18 : Subsystem  AncestorBlock=casper_library/Delays/pipeline  mask(pipeline){latency=1}
      mask help:
      | An explicitly laid-out delay line to avoid mapping to SRL16s
      | for use in pipelining to help achieve timing closure.
      mask init:
      | pipeline_init(gcb, 'latency', latency);
      mask Display:
      | port_label('input', 1, 'd');
      | port_label('output', 1, 'q');
      | disp(['Z^-', num2str(latency)]);
  Delay19 : Subsystem  AncestorBlock=casper_library/Delays/pipeline  mask(pipeline){latency=1}
      mask help:
      | An explicitly laid-out delay line to avoid mapping to SRL16s
      | for use in pipelining to help achieve timing closure.
      mask init:
      | pipeline_init(gcb, 'latency', latency);
      mask Display:
      | port_label('input', 1, 'd');
      | port_label('output', 1, 'q');
      | disp(['Z^-', num2str(latency)]);
  Delay2 : xbsIndex_r4/Delay  rst=off  infoeditControl=Selection of Reset will increase slice count due to use of real FFs and instead of SRLs  en=off  latency=2  dbl_ovrd=off  reg_retiming=off  block_type=delay
  Delay20 : Subsystem  AncestorBlock=casper_library/Delays/pipeline  mask(pipeline){latency=1}
      mask help:
      | An explicitly laid-out delay line to avoid mapping to SRL16s
      | for use in pipelining to help achieve timing closure.
      mask init:
      | pipeline_init(gcb, 'latency', latency);
      mask Display:
      | port_label('input', 1, 'd');
      | port_label('output', 1, 'q');
      | disp(['Z^-', num2str(latency)]);
  Delay22 : Subsystem  AncestorBlock=casper_library/Delays/pipeline  mask(pipeline){latency=1}
      mask help:
      | An explicitly laid-out delay line to avoid mapping to SRL16s
      | for use in pipelining to help achieve timing closure.
      mask init:
      | pipeline_init(gcb, 'latency', latency);
      mask Display:
      | port_label('input', 1, 'd');
      | port_label('output', 1, 'q');
      | disp(['Z^-', num2str(latency)]);
  Delay23 : Subsystem  AncestorBlock=casper_library/Delays/pipeline  mask(pipeline){latency=1}
      mask help:
      | An explicitly laid-out delay line to avoid mapping to SRL16s
      | for use in pipelining to help achieve timing closure.
      mask init:
      | pipeline_init(gcb, 'latency', latency);
      mask Display:
      | port_label('input', 1, 'd');
      | port_label('output', 1, 'q');
      | disp(['Z^-', num2str(latency)]);
  Delay24 : Subsystem  AncestorBlock=casper_library/Delays/pipeline  mask(pipeline){latency=2}
      mask help:
      | An explicitly laid-out delay line to avoid mapping to SRL16s
      | for use in pipelining to help achieve timing closure.
      mask init:
      | pipeline_init(gcb, 'latency', latency);
      mask Display:
      | port_label('input', 1, 'd');
      | port_label('output', 1, 'q');
      | disp(['Z^-', num2str(latency)]);
  Delay25 : Subsystem  AncestorBlock=casper_library/Delays/pipeline  mask(pipeline){latency=1}
      mask help:
      | An explicitly laid-out delay line to avoid mapping to SRL16s
      | for use in pipelining to help achieve timing closure.
      mask init:
      | pipeline_init(gcb, 'latency', latency);
      mask Display:
      | port_label('input', 1, 'd');
      | port_label('output', 1, 'q');
      | disp(['Z^-', num2str(latency)]);
  Delay26 : Subsystem  AncestorBlock=casper_library/Delays/pipeline  mask(pipeline){latency=1}
      mask help:
      | An explicitly laid-out delay line to avoid mapping to SRL16s
      | for use in pipelining to help achieve timing closure.
      mask init:
      | pipeline_init(gcb, 'latency', latency);
      mask Display:
      | port_label('input', 1, 'd');
      | port_label('output', 1, 'q');
      | disp(['Z^-', num2str(latency)]);
  Delay27 : Subsystem  AncestorBlock=casper_library/Delays/pipeline  mask(pipeline){latency=1}
      mask help:
      | An explicitly laid-out delay line to avoid mapping to SRL16s
      | for use in pipelining to help achieve timing closure.
      mask init:
      | pipeline_init(gcb, 'latency', latency);
      mask Display:
      | port_label('input', 1, 'd');
      | port_label('output', 1, 'q');
      | disp(['Z^-', num2str(latency)]);
  Delay3 : Subsystem  AncestorBlock=casper_library/Delays/pipeline  mask(pipeline){latency=1}
      mask help:
      | An explicitly laid-out delay line to avoid mapping to SRL16s
      | for use in pipelining to help achieve timing closure.
      mask init:
      | pipeline_init(gcb, 'latency', latency);
      mask Display:
      | port_label('input', 1, 'd');
      | port_label('output', 1, 'q');
      | disp(['Z^-', num2str(latency)]);
  Delay44 : Subsystem  AncestorBlock=casper_library/Delays/pipeline  mask(pipeline){latency=2}
      mask help:
      | An explicitly laid-out delay line to avoid mapping to SRL16s
      | for use in pipelining to help achieve timing closure.
      mask init:
      | pipeline_init(gcb, 'latency', latency);
      mask Display:
      | port_label('input', 1, 'd');
      | port_label('output', 1, 'q');
      | disp(['Z^-', num2str(latency)]);
  Delay46 : Subsystem  AncestorBlock=casper_library/Delays/pipeline  mask(pipeline){latency=2}
      mask help:
      | An explicitly laid-out delay line to avoid mapping to SRL16s
      | for use in pipelining to help achieve timing closure.
      mask init:
      | pipeline_init(gcb, 'latency', latency);
      mask Display:
      | port_label('input', 1, 'd');
      | port_label('output', 1, 'q');
      | disp(['Z^-', num2str(latency)]);
  Delay76 : Subsystem  AncestorBlock=casper_library/Delays/pipeline  mask(pipeline){latency=2}
      mask help:
      | An explicitly laid-out delay line to avoid mapping to SRL16s
      | for use in pipelining to help achieve timing closure.
      mask init:
      | pipeline_init(gcb, 'latency', latency);
      mask Display:
      | port_label('input', 1, 'd');
      | port_label('output', 1, 'q');
      | disp(['Z^-', num2str(latency)]);
  Delay79 : Subsystem  AncestorBlock=casper_library/Delays/pipeline  mask(pipeline){latency=2}
      mask help:
      | An explicitly laid-out delay line to avoid mapping to SRL16s
      | for use in pipelining to help achieve timing closure.
      mask init:
      | pipeline_init(gcb, 'latency', latency);
      mask Display:
      | port_label('input', 1, 'd');
      | port_label('output', 1, 'q');
      | disp(['Z^-', num2str(latency)]);
  Register0 : xbsIndex_r4/Register  init=1  rst=off  en=off  dbl_ovrd=off  block_type=register
  Register1 : xbsIndex_r4/Register  init=1  rst=off  en=off  dbl_ovrd=off  block_type=register
  Subsystem1 : Subsystem
  Subsystem12 : Subsystem
  loop_cnt : xps_library/software register  Tag=xps:sw_reg  SystemSampleTime=-1  io_dir=To Processor  arith_type=Unsigned  bitwidth=32  bin_pt=0  sample_period=1  gw_name=roachf_1024_bao_loopback_loop_cnt_user_data_in
      link override convert: arith_type=Unsigned  n_bits=32  bin_pt=0
  loop_err_cnt : xps_library/software register  Tag=xps:sw_reg  SystemSampleTime=-1  io_dir=To Processor  arith_type=Unsigned  bitwidth=32  bin_pt=0  sample_period=1  gw_name=roachf_1024_bao_loopback_loop_err_cnt_user_data_in
      link override convert: arith_type=Unsigned  n_bits=32  bin_pt=0
  loopback mux : Subsystem
  loopback_fifo : Subsystem
  rx_cnt : xps_library/software register  Tag=xps:sw_reg  SystemSampleTime=-1  io_dir=To Processor  arith_type=Unsigned  bitwidth=32  bin_pt=0  sample_period=1  gw_name=roachf_1024_bao_loopback_rx_cnt_user_data_in
      link override convert: arith_type=Unsigned  n_bits=32  bin_pt=0
  rx_err_cnt : xps_library/software register  Tag=xps:sw_reg  SystemSampleTime=-1  io_dir=To Processor  arith_type=Unsigned  bitwidth=32  bin_pt=0  sample_period=1  gw_name=roachf_1024_bao_loopback_rx_err_cnt_user_data_in
      link override convert: arith_type=Unsigned  n_bits=32  bin_pt=0
  rx_pkt_fifo : Subsystem
      settings: AttributesFormatString=|
      | Max 1024 data words.
      | Max 32 pkts.
  Out1 : Outport
  tag scope: lb_mux_data=global, lb_mux_eof=global, lb_mux_header=global, lb_mux_valid=global
  wires:
  [cnt_rst] -> Delay8/1
  Subsystem12/2(err_cnt) -> loop_err_cnt/1
  Subsystem12/1(rx_cnt) -> loop_cnt/1
  [loopback_mux_rst] -> loopback mux/1(rst)
  [gbe_sw_rx_valid] -> Delay76/1(d)
  [gbe_sw_rx] -> Delay79/1(d)
  [gbe_sw_eof] -> Delay24/1(d)
  Delay79/1(q) -> rx_pkt_fifo/1(d_in)
  Delay76/1(q) -> rx_pkt_fifo/2(valid_in)
  Delay24/1(q) -> rx_pkt_fifo/3(eof_in)
  [my_ip] -> Delay46/1(d)
  [gbe_sw_tx_data] -> Delay14/1(d)
  [gbe_sw_valid_tx] -> Delay15/1(d)
  [gbe_sw_tx_ip] -> Delay16/1(d)
  [gbe_sw_tx_eof] -> Delay44/1(d)
  Delay14/1(q) -> loopback_fifo/1(din)
  Delay15/1(q) -> loopback_fifo/2(we)
  Delay16/1(q) -> loopback_fifo/3(dest_ip)
  Delay44/1(q) -> loopback_fifo/4(eof)
  Delay46/1(q) -> loopback_fifo/5(my_ip)
  In1/1 -> Out1/1
  Delay1/1 -> loopback_fifo/6(re)
  Subsystem1/1(rx_cnt) -> rx_cnt/1
  Subsystem1/2(err_cnt) -> rx_err_cnt/1
  rx_pkt_fifo/1(data) -> Delay3/1(d)
  rx_pkt_fifo/2(valid) -> Delay5/1, Delay17/1(d)
  rx_pkt_fifo/3(eof) -> Delay6/1, Delay18/1(d)
  rx_pkt_fifo/4(wr_ack) -> Delay19/1(d)
  rx_pkt_fifo/5(full) -> Delay7/1, Delay20/1(d)
  rx_pkt_fifo/6(empty) -> Register1/1
  loopback_fifo/1(dout) -> Delay22/1(d)
  loopback_fifo/2(valid) -> Delay9/1, Delay23/1(d)
  loopback_fifo/3(eof_out) -> Delay10/1, Delay25/1(d)
  loopback_fifo/4(wr_ack) -> Delay26/1(d)
  loopback_fifo/5(full) -> Delay11/1, Delay27/1(d)
  loopback_fifo/6(empty) -> Register0/1
  [cnt_rst] -> Delay4/1
  loopback mux/1(dout) -> [lb_mux_data]
  loopback mux/2(valid_out) -> [lb_mux_valid]
  loopback mux/3(eof) -> [lb_mux_eof]
  loopback mux/4(header_out) -> [lb_mux_header]
  loopback mux/5(gbe_read) -> [gbe_read]
  loopback mux/6(loop_read) -> [loop_read]
  Delay2/1 -> rx_pkt_fifo/4(re)
  [gbe_read] -> Delay2/1
  [loop_read] -> Delay1/1
  Delay4/1 -> Subsystem1/1(rst)
  Delay5/1 -> Subsystem1/2(we)
  Delay6/1 -> Subsystem1/3(eof)
  Delay7/1 -> Subsystem1/4(overflow)
  Delay8/1 -> Subsystem12/1(rst)
  Delay9/1 -> Subsystem12/2(we)
  Delay10/1 -> Subsystem12/3(eof)
  Delay11/1 -> Subsystem12/4(overflow)
  Delay3/1(q) -> loopback mux/2(gbe_din)
  Delay17/1(q) -> loopback mux/3(gbe_valid)
  Delay18/1(q) -> loopback mux/4(gbe_eof)
  Delay19/1(q) -> loopback mux/5(gbe_wr_ack)
  Delay20/1(q) -> loopback mux/6(gbe_full)
  Register1/1 -> loopback mux/7(gbe_empty)
  Delay22/1(q) -> loopback mux/8(loop_din)
  Delay23/1(q) -> loopback mux/9(loop_valid)
  Delay25/1(q) -> loopback mux/10(loop_eof)
  Delay26/1(q) -> loopback mux/11(loop_wr_ack)
  Delay27/1(q) -> loopback mux/12(loop_full)
  Register0/1 -> loopback mux/13(loop_empty)

== system roachf_1024_bao/seed ==
  BitBasher : xbsIndex_r4/BitBasher  bitexpr=|  display_expr=off  sr_1=1  arith_type1=Unsigned  bin_pt1=0  sr_2=2  arith_type2=Unsigned  bin_pt2=0  sr_3=3  arith_type3=Unsigned  bin_pt3=0  sr_4=4  arith_type4=Unsigned  bin_pt4=0  dbl_ovrd=off  block_type=bitbasher
      | <html><head><meta name="qrichtext" content="1" /><style type="text/css">
      | p, li { white-space: pre-wrap; }
      | </style></head><body style=" font-family:'MS Shell Dlg 2'; font-size:8.25pt; font-weight:400; font-style:normal;">
      | <p style=" margin-top:12px; margin-bottom:12px; margin-left:0px; margin-right:0px; -qt-block-indent:0; text-indent:0px; font-family:'MS Shell Dlg'; font-size:8pt;">seed0={8'h5c, seed[7:0], seed[0:7], 8'ha3}<br />seed1={8'h5c, seed[15:8], seed[8:15], 8'ha3}<br />seed2={8'h5c, seed[23:16], seed[16:23], 8'ha3}<br />seed3={8'h5c, seed[31:24], seed[24:31], 8'ha3}</p></body></html>
      settings: block_version=10.1.3
  armed_trigger : casper_library_misc/armed_trigger  SystemSampleTime=-1  hidden=0
  data : xps_library/software register  Tag=xps:sw_reg  SystemSampleTime=-1  io_dir=From Processor  arith_type=Unsigned  bitwidth=32  bin_pt=0  sample_period=1  gw_name=roachf_1024_bao_seed_data_user_data_out
  tag scope: seed0=global, seed1=global, seed2=global, seed3=global, seed_ld=global
  wires:
  [arm_rst] -> armed_trigger/1
  data/1 -> BitBasher/1
  [sync_gen] -> armed_trigger/2
  armed_trigger/1 -> [seed_ld]
  BitBasher/4 -> [seed3]
  BitBasher/3 -> [seed2]
  BitBasher/2 -> [seed1]
  BitBasher/1 -> [seed0]
